simulink model "unicycle_polar_on_spot_simulink"  (R2020b)
settings: Solver=VariableStepAuto  StartTime=0.0  StopTime=100  RelTol=1e-3
values from neighbouring files (symbols this model uses):
  Current_coordinates = Target_coordinates    [checking_simulink_with_matlab.m]    (also in lloyd_wtd_adaptive_nonconvex.m = [Prev_Px(i); Prev_Py(i)]; lloyd_wtd_unicycle.m = [Prev_Px(i); Prev_Py(i)])
  init_heading = b(end)    [checking_simulink_with_matlab.m]    (also in lloyd_wtd_adaptive_nonconvex.m = init_heading_list(i); lloyd_wtd_unicycle.m = init_heading_list(i))
  Target_coordinates = [round(rand(1)*10);round(rand(1)*10) ]    [checking_simulink_with_matlab.m]    (also in lloyd_wtd_adaptive_nonconvex.m = [Px(i);Py(i)]; lloyd_wtd_unicycle.m = [Px(i);Py(i)])
libraries: simulink x3, robotmobilelib x1
settings Model: SimulationMode=accelerator  Creator=nijil  LastModifiedBy=nijil

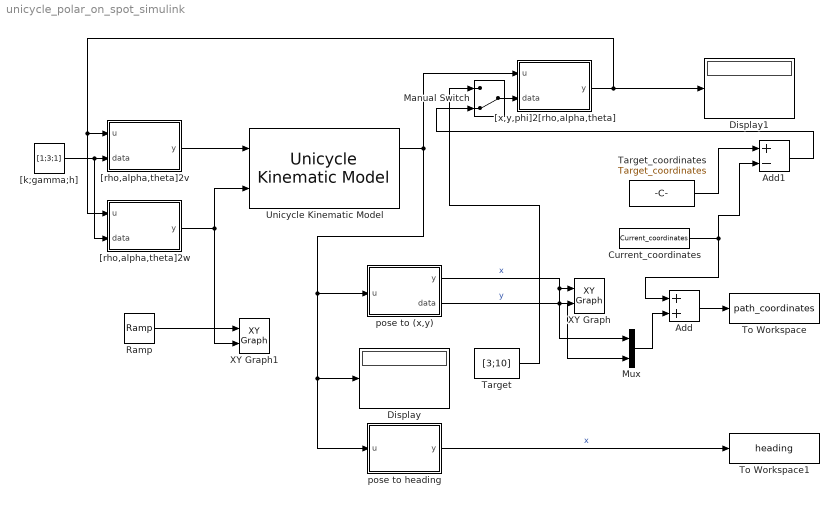
== system unicycle_polar_on_spot_simulink ==
  Add : Sum
  Add1 : Sum  Inputs=+-
  Current_coordinates : Constant  Value=Current_coordinates
  Display : Display
  Display1 : Display
  Manual Switch : ManualSwitch  CurrentSetting=0
  Mux : Mux  Inputs=2
  Ramp : simulink/Sources/Ramp  slope=1  start=0  InitialOutput=0
  Target : Constant  Value=[3;10]  VectorParams1D=off
  Target_coordinates : Constant  Value=Target_coordinates
  To Workspace : ToWorkspace  VariableName=path_coordinates  SaveFormat=Timeseries  SampleTime=-1
  To Workspace1 : ToWorkspace  VariableName=heading  SaveFormat=Timeseries  SampleTime=-1
  Unicycle Kinematic Model : robotmobilelib/Unicycle Kinematic Model  VehicleInputs=Vehicle Speed & Heading Angular Velocity  WheelRadius=0.1  WheelSpeedRange=[-pi pi]  InitialState=[0 0 init_heading]  SimulateUsing=Interpreted execution
      settings: SourceProductBaseCode=RO
  XY Graph : simulink/Sinks/XY Graph  xmin=-10  xmax=10  ymin=-10  ymax=10  st=-1
  XY Graph1 : simulink/Sinks/XY Graph  xmin=0  xmax=50  ymin=-10  ymax=10  st=-1
  "[k;gamma;h]" : Constant  Value=[1;3;1]  VectorParams1D=off
  "[rho,alpha,theta]2v" : MATLAB Function  TreatAsAtomicUnit=on
  "[rho,alpha,theta]2w" : MATLAB Function  TreatAsAtomicUnit=on
  "[x,y,phi]2[rho,alpha,theta]" : MATLAB Function  TreatAsAtomicUnit=on
  pose to (x,y) : MATLAB Function  TreatAsAtomicUnit=on
  pose to heading : MATLAB Function  TreatAsAtomicUnit=on
  wires:
  "[rho,alpha,theta]2v"/1(y) -> Unicycle Kinematic Model/1
  Unicycle Kinematic Model/1 -> "[x,y,phi]2[rho,alpha,theta]"/1(u), pose to heading/1(u), Display/1, pose to (x,y)/1(u)
  "[k;gamma;h]"/1 -> "[rho,alpha,theta]2w"/2(data), "[rho,alpha,theta]2v"/2(data)
  pose to (x,y)/1(y) -> Mux/1, XY Graph/1  "x"
  pose to (x,y)/2(data) -> Mux/2, XY Graph/2  "y"
  Target/1 -> Manual Switch/1
  "[x,y,phi]2[rho,alpha,theta]"/1(y) -> Display1/1, "[rho,alpha,theta]2w"/1(u), "[rho,alpha,theta]2v"/1(u)
  "[rho,alpha,theta]2w"/1(y) -> XY Graph1/2, Unicycle Kinematic Model/2
  Ramp/1 -> XY Graph1/1
  Manual Switch/1 -> "[x,y,phi]2[rho,alpha,theta]"/2(data)
  Target_coordinates/1 -> Add1/1
  Current_coordinates/1 -> Add1/2, Add/1
  Add/1 -> To Workspace/1
  Mux/1 -> Add/2
  Add1/1 -> Manual Switch/2
  pose to heading/1(y) -> To Workspace1/1  "x"

== matlab function unicycle_polar_on_spot_simulink/[rho,alpha,theta]2v ==
  data: u input; y output; data input
function y = fcn(u, data)
%data=[k;gamma;h], u=[rho,alpha,theta]
if u(2)>0
    y = data(2)*cos(u(2))*u(1);
else
    y=data(2)*cos(u(2))*u(1);
end

== matlab function unicycle_polar_on_spot_simulink/pose to (x,y) ==
  data: u input; y output; data output
function [y,data] = fcn(u)
y=u(1);
data = u(2);

== matlab function unicycle_polar_on_spot_simulink/[x,y,phi]2[rho,alpha,theta] ==
  data: u input; y output; data input
function y = fcn(u, data)
%u=[x;y;phi], data=[x_c;y_c], y=[rho,alpha,theta]
rho=sqrt((u(1)-data(1))^2+(u(2)-data(2))^2);
alpha=-u(3)+atan2((data(2)-u(2)),(data(1)-u(1)));
theta=atan2((data(2)-u(2)),(data(1)-u(1)));
y =[rho;alpha;theta];

== matlab function unicycle_polar_on_spot_simulink/pose to heading ==
  data: u input; y output
function y = fcn(u)

y = u(3);

== matlab function unicycle_polar_on_spot_simulink/[rho,alpha,theta]2w ==
  data: u input; y output; data input
function y = fcn(u, data)
%data=[k;gamma;h], u=[rho,alpha,theta]
y =2*data(1)*u(2)+data(2)*cos(u(2))*sin(u(2))*(u(2)+data(3)*u(3))/u(2);
